simulink model "EMG_DR_E2E_pipeline_simulink"  (R2025a)
settings: Solver=FixedStepAuto  StartTime=0.0  StopTime=inf  FixedStep=0.001  RelTol=1e-3
undefined symbols (not defined in the file or in its folder): magnitude
libraries: slpidlib x4, instrumentseriallib x2, sim3dlib x1, uavsim3dlib x1, deeplib x1
settings Model: Creator=user  LastModifiedBy=82102

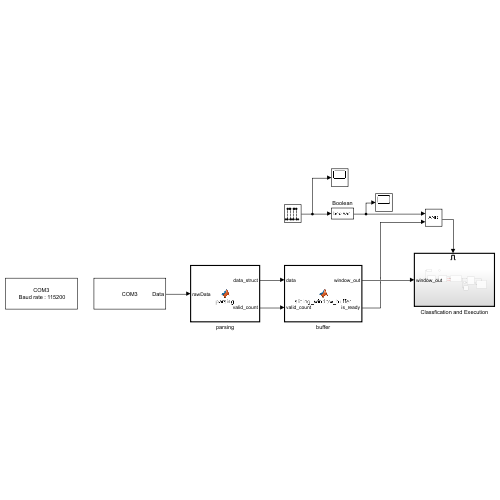
[thumbnail: Simulink's stored preview of the top-level diagram]
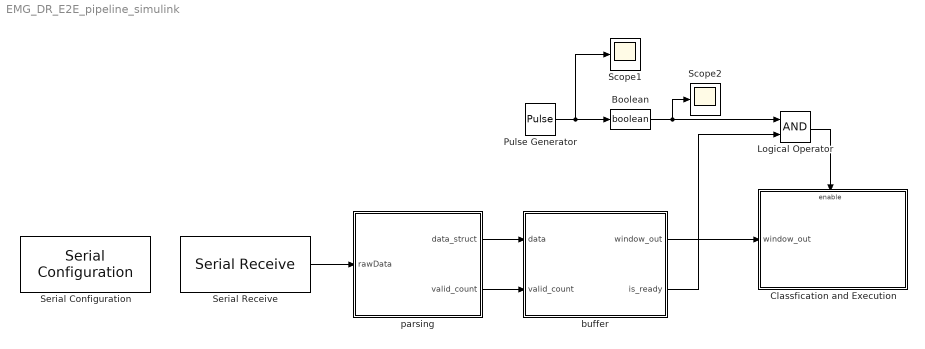
== system EMG_DR_E2E_pipeline_simulink ==
  Boolean : DataTypeConversion  OutDataTypeStr=boolean  SaturateOnIntegerOverflow=off  RndMeth=Floor
  Classfication and Execution : Subsystem  TreatAsAtomicUnit=on
  Logical Operator : Logic  AllPortsSameDT=off  OutDataTypeStr=boolean
  Pulse Generator : DiscretePulseGenerator  Period=100  SampleTime=0.001
  Scope1 : Scope
      settings: ActiveDisplayYMinimum=-1.4E-5  ActiveDisplayYMaximum=1.9E-5
  Scope2 : Scope
      settings: ActiveDisplayYMinimum=-2.3E-6  ActiveDisplayYMaximum=2.1E-6  DataLoggingVariableName=ScopeData2
  Serial Configuration : instrumentseriallib/Serial Configuration  Priority=-200000  PortSel=COM3  Port=COM3  ComPort=COM3  BaudRate=115200  DataBits=8  Parity=none  StopBits=1  ByteOrder=little-endian  FlowControl=none  Timeout=10  SimulateUsing=Interpreted execution  BlockInModel=on  aMode=1
  Serial Receive : instrumentseriallib/Serial Receive  Priority=1  PortSel=COM3  Port=COM3  ComPort=COM3  DataType=uint8  SaveDataType=uint8  ToggleHeader=off  Header=[]  ToggleDataSize=on  DataSize=[1 27]  ToggleTerminator=off  Terminator=<none>  CustomTerminator=[]  InputFormat=Column major  EnableBlockingMode=on  ActionDataUnavailable=Output last received value  ActionWhenDataUnavailable=Output last received value  CustomValue=0  SampleTime=0.001  SimulateUsing=Interpreted execution  BlockInModel=on  aMode=1  LibraryInUse=instrumentlib
  buffer : MATLAB Function  TreatAsAtomicUnit=on
  parsing : MATLAB Function  TreatAsAtomicUnit=on  SystemSampleTime=0.001
  wires:
  Serial Receive/1 -> parsing/1(rawData)
  parsing/1(data_struct) -> buffer/1(data)
  parsing/2(valid_count) -> buffer/2(valid_count)
  Pulse Generator/1 -> Boolean/1, Scope1/1
  Boolean/1 -> Logical Operator/1, Scope2/1
  buffer/1(window_out) -> Classfication and Execution/1(window_out)
  Logical Operator/1 -> Classfication and Execution/Enable
  buffer/2(is_ready) -> Logical Operator/2

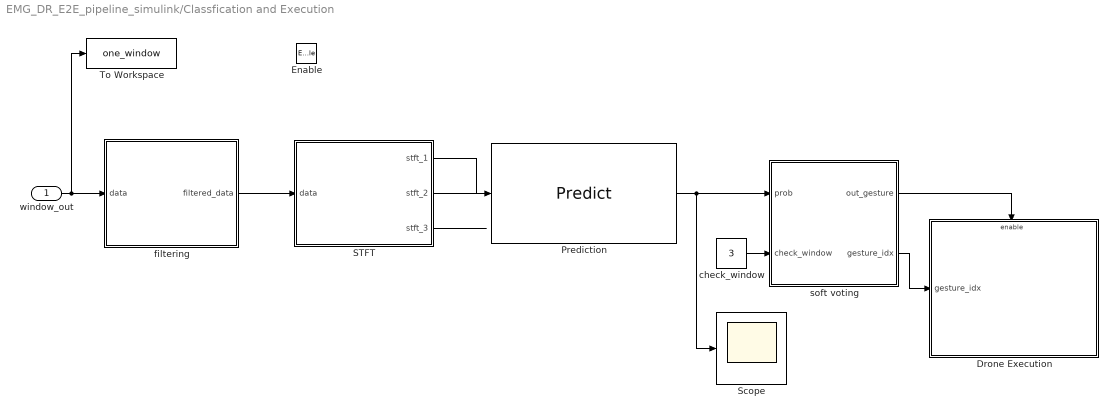
== system EMG_DR_E2E_pipeline_simulink/Classfication and Execution ==
  window_out : Inport
  Enable : EnablePort
  Drone Execution : Subsystem  TreatAsAtomicUnit=on
  Prediction : deeplib/Predict  Network=Network from MAT-file  NetworkFunction=squeezenet  NetworkFilePath=C:\Users\user\Desktop\MATLAB\model\trained_model_3ch_lstm.mat  MiniBatchSize=1  InputDataFormats={'',''}  Predictions=on  Activations={}  ForceInterpretedSim=off  EnableDLNetwork=on  LastKnownNetworkFilePath=''  LastKnownNetworkTimeStamp=''
  STFT : MATLAB Function  TreatAsAtomicUnit=on
  Scope : Scope
      settings: ActiveDisplayYMinimum=-0.125  ActiveDisplayYMaximum=1.125
  To Workspace : ToWorkspace  VariableName=one_window  SampleTime=-1
  check_window : Constant  Value=3
  filtering : MATLAB Function  TreatAsAtomicUnit=on
  soft voting : MATLAB Function  TreatAsAtomicUnit=on
  wires:
  check_window/1 -> soft voting/2(check_window)
  filtering/1(filtered_data) -> STFT/1(data)
  STFT/1(stft_1) -> Prediction/1
  Prediction/1 -> soft voting/1(prob), Scope/1
  window_out/1 -> To Workspace/1, filtering/1(data)
  soft voting/1(out_gesture) -> Drone Execution/Enable
  soft voting/2(gesture_idx) -> Drone Execution/1(gesture_idx)
  STFT/2(stft_2) -> ?
  STFT/3(stft_3) -> ?

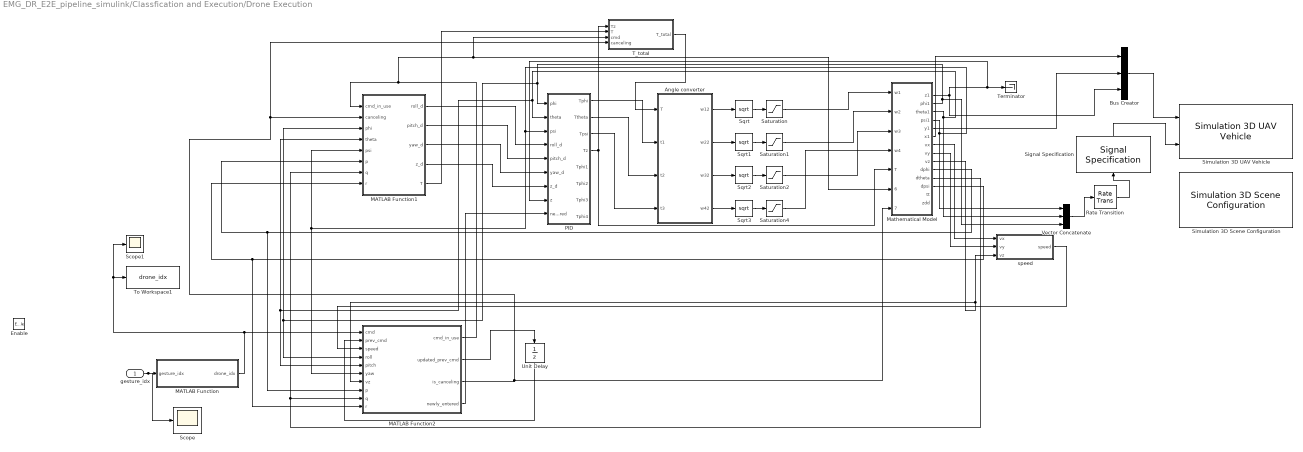
== system EMG_DR_E2E_pipeline_simulink/Classfication and Execution/Drone Execution ==
  gesture_idx : Inport
  Enable : EnablePort
  Angle converter : MATLAB Function  TreatAsAtomicUnit=on
  Bus Creator : BusCreator  Inputs=3
  MATLAB Function : MATLAB Function  TreatAsAtomicUnit=on
  MATLAB Function1 : MATLAB Function  TreatAsAtomicUnit=on
  MATLAB Function2 : MATLAB Function  TreatAsAtomicUnit=on
  Mathematical Model : Subsystem
  PID : Subsystem
  Rate Transition : RateTransition  Deterministic=off  OutPortSampleTime=0.01
  Saturation{,1..2,4} (4 alike) : Saturate  UpperLimit=8000  LowerLimit=0
  Scope : Scope
  Scope1 : Scope
      settings: ActiveDisplayYMinimum=0  ActiveDisplayYMaximum=9
  Signal Specification : SignalSpecification  OutDataTypeStr=double  Dimensions=[1 3]  SampleTime=0.01
  Simulation 3D Scene Configuration : sim3dlib/Simulation 3D Scene Configuration  Priority=0  ProjectFormat=Default Scenes  SceneDesc=US city block  ProjectName=C:\Program Files\MATLAB\R2025a\toolbox\shared\sim3d_projects\automotive_project_windows\UE\WindowsNoEditor\VehicleSimulation.exe  ScenePath=/Game/Maps/USCityBlock  EnableOpenDRIVE=off  vehTagList={'Scene Origin'}  vehTag=Scene Origin  AttachedCameraRelativeTranslation=[0 0 0]  FreeCameraDefaultInitialTranslation=[-6, 0, 2]  AttachedCameraRelativeRotation=[0 0 0]  FreeCameraDefaultInitialRotation=[0, -15, 0]  ViewpointName=Custom  FreeCameraInitialTranslation=[0, 0, 0]  ViewpointTranslation=[0 0 0]  FreeCameraInitialRotation=[0, 0, 0]  ViewpointRotation=[0 0 0]  OpVisEn=off  Ts=0.01  EnableWindow=on  EnableRemoteAccess=off  EnableWeather=off  SunAzimuth=90  SunAltitude=40.0  EnableGeospatialSun=off  Latitude=0  Longitude=0  Date=2023-01-01  Time=10:30:00  GeoTimeZone=-5.0  SunDaylightSaving=off  wind=1  clouds=10  EnableVolumetricClouds=off  CloudCoverage=0  CloudAltitude=6  fog=0  rain=0  RaindropsEffect=off  SnowDensity=0  EnableGeospatial=off  TilesetSource=Earth terrain  UseTrueOrigin=off  OriginHeight=200  OriginLatitude=40.744652  OriginLongitude=-73.988864  MapStyle=Aerial  AdditionalAssetIDs=[]  UseAdvancedSunSky=off  SolarTime=11  TimeZone=-5  Day=21  Month=9  Year=2022  UseDaylightSavingTime=on  DSTStartDay=10  DSTStartMonth=3  DSTEndDay=3  DSTEndMonth=11  DSTSwitchHour=2  sensorTag=MainCamera1  sensorId=1  sensorName=MainCamera1  mountLoc=Origin  offsetFlag=off  tmountOffset=[0, 0, 0]  rmountOffset=[0, 0, 0]  HorizontalResolution=1280  VerticalResolution=720  HorizontalFOV=60  mountPoint=[0 0 0]  mountOrientation=[0 0 0]  aMode=4  ID=1  GeoTrigger=Inactive  ViewNameList={'Custom'}  ViewTranslationList={'[0 0 0]'}  ViewRotationList={'[0 0 0]'}
      settings: LibrarySourceBlock=uavsim3dlib/Simulation 3D Scene Configuration
  Simulation 3D UAV Vehicle : uavsim3dlib/Simulation 3D UAV Vehicle  Priority=-1  Mesh=Quadrotor  MeshPath=/MathWorksUAVContent/UAVs/HexaRotorUAV/HexaRotor.HexaRotor  Color=Red  ActorName=SimulinkVehicle1  UseGlobalFrame=off  InitialTranslation=[0 0 0]  InitialRotation=[0 0 0]  InitialTranslationGlobal=[0 0 0]  InitialGeoOrigin=[0 0 0]  InitialRotationGlobal=[0 0 0]  SampleTime=0.01  ActorType=SimulinkVehicle  ID=1  aMode=4  ActorTag=SimulinkVehicle1
  Sqrt{,1..3} (4 alike) : Sqrt
  T_total : MATLAB Function  TreatAsAtomicUnit=on
  Terminator : Terminator
  To Workspace1 : ToWorkspace  VariableName=drone_idx  SaveFormat=Timeseries  SampleTime=-1
      settings: Save2DSignal=2-D array (concatenate along first dimension)
  Unit Delay : UnitDelay  SampleTime=-1  HasFrameUpgradeWarning=on
  Vector Concatenate : Concatenate  NumInputs=3
  speed : Subsystem
  wires:
  Saturation1/1 -> Mathematical Model/2(w2)
  Angle converter/3(w32) -> Sqrt2/1
  PID/3(Tpsi) -> Angle converter/4(t3)
  Vector Concatenate/1 -> Rate Transition/1
  MATLAB Function1/1(roll_d) -> PID/4(roll_d)
  Bus Creator/1 -> Simulation 3D UAV Vehicle/1
  Mathematical Model/9(vz) -> MATLAB Function2/7(vz), speed/3(vz)
  Mathematical Model/5(y1) -> Bus Creator/2
  MATLAB Function2/1(cmd_in_use) -> MATLAB Function1/1(cmd_in_use), T_total/3(cmd), Mathematical Model/6(cmd_in_use)
  MATLAB Function1/5(T) -> T_total/2(T)
  speed/1(speed) -> MATLAB Function2/3(speed)
  Sqrt2/1 -> Saturation2/1
  Angle converter/2(w22) -> Sqrt1/1
  Saturation/1 -> Mathematical Model/1(w1)
  Mathematical Model/7(vx) -> speed/1(vx)
  PID/2(Ttheta) -> Angle converter/3(t2)
  Saturation4/1 -> Mathematical Model/4(w4)
  MATLAB Function2/3(is_canceling) -> T_total/4(canceling), MATLAB Function1/2(canceling), Mathematical Model/7(is_canceling)
  Saturation2/1 -> Mathematical Model/3(w3)
  MATLAB Function2/2(updated_prev_cmd) -> Unit Delay/1
  Mathematical Model/8(vy) -> speed/2(vy)
  Sqrt/1 -> Saturation/1
  Mathematical Model/6(x1) -> Bus Creator/1
  PID/1(Tphi) -> Angle converter/2(t1)
  MATLAB Function1/3(yaw_d) -> PID/6(yaw_d)
  Angle converter/1(w12) -> Sqrt/1
  Sqrt3/1 -> Saturation4/1
  Signal Specification/1 -> Simulation 3D UAV Vehicle/2
  MATLAB Function2/4(newly_entered) -> PID/9(newly_entered)
  MATLAB Function1/2(pitch_d) -> PID/5(pitch_d)
  Mathematical Model/12(dpsi) -> MATLAB Function1/8(r), MATLAB Function2/10(r)
  Rate Transition/1 -> Signal Specification/1
  Sqrt1/1 -> Saturation1/1
  T_total/1(T_total) -> Angle converter/1(T)
  Angle converter/4(w42) -> Sqrt3/1
  Mathematical Model/1(z1) -> PID/8(z), Terminator/1, Bus Creator/3
  Mathematical Model/3(theta1) -> Vector Concatenate/2, PID/2(theta), MATLAB Function1/4(theta), MATLAB Function2/5(pitch)
  Mathematical Model/4(psi1) -> Vector Concatenate/1, MATLAB Function1/5(psi), MATLAB Function2/6(yaw), PID/3(psi)
  Mathematical Model/10(dphi) -> MATLAB Function1/6(p), MATLAB Function2/8(p)
  Mathematical Model/2(phi1) -> MATLAB Function1/3(phi), MATLAB Function2/4(roll), PID/1(phi), Vector Concatenate/3
  MATLAB Function1/4(z_d) -> PID/7(z_d)
  PID/4(Tz) -> T_total/1(Tz), Mathematical Model/5(T)
  Unit Delay/1 -> MATLAB Function2/2(prev_cmd)
  Mathematical Model/11(dtheta) -> MATLAB Function2/9(q), MATLAB Function1/7(q)
  gesture_idx/1 -> Scope/1, MATLAB Function/1(gesture_idx)
  MATLAB Function/1(drone_idx) -> MATLAB Function2/1(cmd), Scope1/1, To Workspace1/1

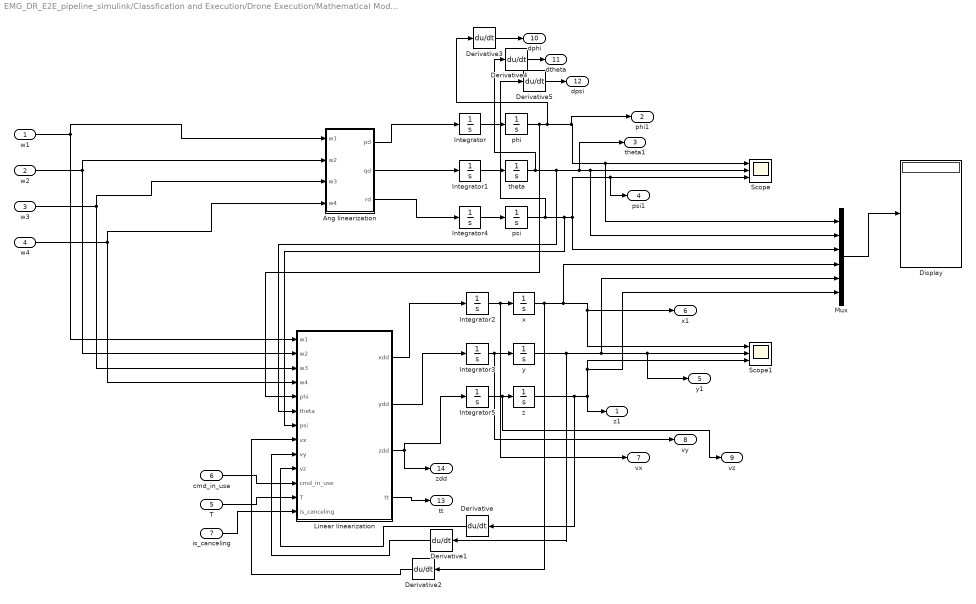
== system EMG_DR_E2E_pipeline_simulink/Classfication and Execution/Drone Execution/Mathematical Model ==
  w1 : Inport
  w2 : Inport  Port=2
  w3 : Inport  Port=3
  w4 : Inport  Port=4
  T : Inport  Port=5
  cmd_in_use : Inport  Port=6
  is_canceling : Inport  Port=7
  Ang linearization : MATLAB Function  TreatAsAtomicUnit=on
  Derivative : Derivative  CoefficientInTFapproximation=0.01
  Derivative1 : Derivative  CoefficientInTFapproximation=0.01
  Derivative2 : Derivative  CoefficientInTFapproximation=0.01
  Derivative3 : Derivative
  Derivative4 : Derivative
  Derivative5 : Derivative
  Display : Display
  Integrator{,1..5} (6 alike) : Integrator
  Linear linearization : MATLAB Function  TreatAsAtomicUnit=on
  Mux : Mux  Inputs=6
  Scope : Scope  NumInputPorts=3
      settings: ActiveDisplayYMinimum=-1  ActiveDisplayYMaximum=1
  Scope1 : Scope  NumInputPorts=3
      settings: ActiveDisplayYMinimum=-3.8299013315849712E+14  ActiveDisplayYMaximum=3.446911198426474E+15
  phi : Integrator
  psi : Integrator
  theta : Integrator
  x : Integrator
  y : Integrator
  z : Integrator
  z1 : Outport
  phi1 : Outport  Port=2
  theta1 : Outport  Port=3
  psi1 : Outport  Port=4
  y1 : Outport  Port=5
  x1 : Outport  Port=6
  vx : Outport  Port=7
  vy : Outport  Port=8
  vz : Outport  Port=9
  dphi : Outport  Port=10
  dtheta : Outport  Port=11
  dpsi : Outport  Port=12
  tt : Outport  Port=13
  zdd : Outport  Port=14
  wires:
  w3/1 -> Ang linearization/3(w3), Linear linearization/3(w3)
  w4/1 -> Ang linearization/4(w4), Linear linearization/4(w4)
  w1/1 -> Ang linearization/1(w1), Linear linearization/1(w1)
  Integrator5/1 -> vz/1, z/1
  Ang linearization/2(qd) -> Integrator1/1
  psi/1 -> Derivative5/1, Linear linearization/7(psi), psi1/1, Scope/3, Mux/3
  Mux/1 -> Display/1
  Integrator4/1 -> psi/1
  w2/1 -> Ang linearization/2(w2), Linear linearization/2(w2)
  Ang linearization/3(rd) -> Integrator4/1
  Linear linearization/2(ydd) -> Integrator3/1
  theta/1 -> Derivative4/1, Linear linearization/6(theta), theta1/1, Mux/2, Scope/2
  Linear linearization/3(zdd) -> Integrator5/1, zdd/1
  phi/1 -> Linear linearization/5(phi), Derivative3/1, phi1/1, Mux/1, Scope/1
  Integrator2/1 -> vx/1, x/1
  Integrator3/1 -> vy/1, y/1
  Linear linearization/1(xdd) -> Integrator2/1
  Integrator1/1 -> theta/1
  x/1 -> Derivative2/1, Mux/4, Scope1/1, x1/1
  z/1 -> Derivative/1, Mux/6, Scope1/3, z1/1
  Ang linearization/1(pd) -> Integrator/1
  Integrator/1 -> phi/1
  y/1 -> Derivative1/1, Mux/5, y1/1, Scope1/2
  Derivative/1 -> Linear linearization/10(vz)
  Derivative1/1 -> Linear linearization/9(vy)
  Derivative2/1 -> Linear linearization/8(vx)
  Linear linearization/4(tt) -> tt/1
  T/1 -> Linear linearization/12(T)
  cmd_in_use/1 -> Linear linearization/11(cmd_in_use)
  is_canceling/1 -> Linear linearization/13(is_canceling)
  Derivative3/1 -> dphi/1
  Derivative4/1 -> dtheta/1
  Derivative5/1 -> dpsi/1

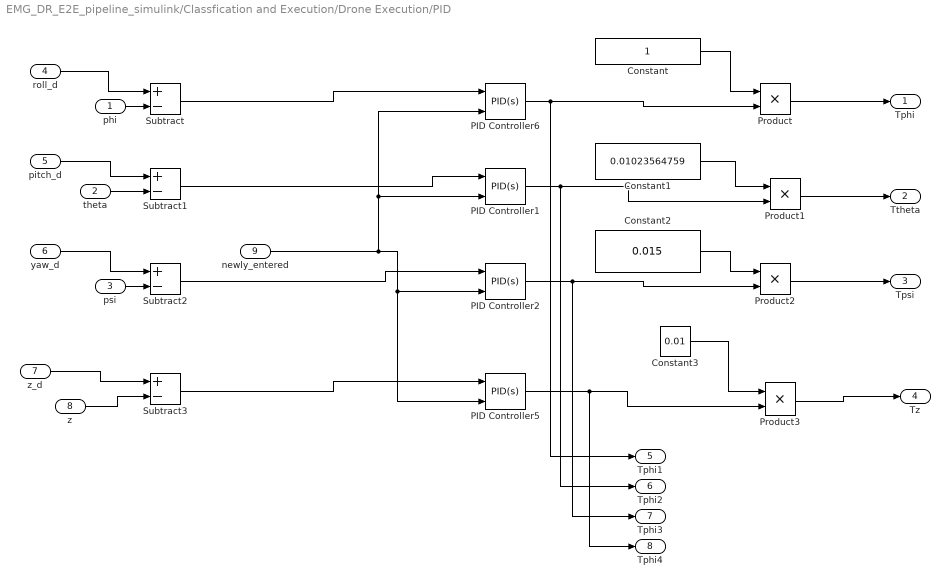
== system EMG_DR_E2E_pipeline_simulink/Classfication and Execution/Drone Execution/PID ==
  phi : Inport
  theta : Inport  Port=2
  psi : Inport  Port=3
  roll_d : Inport  Port=4
  pitch_d : Inport  Port=5
  yaw_d : Inport  Port=6
  z_d : Inport  Port=7
  z : Inport  Port=8
  newly_entered : Inport  Port=9
  Constant : Constant
  Constant1 : Constant  Value=0.01023564759
  Constant2 : Constant  Value=0.015
  Constant3 : Constant  Value=0.01
  PID Controller1 : slpidlib/PID Controller  Controller=PID  Form=Parallel  TimeDomain=Continuous-time  UseExternalTs=off  SampleTime=-1  IntegratorMethod=Forward Euler  FilterMethod=Forward Euler  ControllerParametersSource=internal  P=4.5  I=0.05  UseKiTs=off  D=0.5  UseExternalDerivativeSource=off  N=100  UseFilter=on  TunerSelectOption=Transfer Function Based (PID Tuner App)  InitialConditionSource=internal  InitialConditionForIntegrator=0  InitialConditionForFilter=0  DifferentiatorICPrevScaledInput=0  ExternalReset=rising  TrackingMode=off  Kt=1  LimitOutput=off  SatLimitsSource=internal  UpperSaturationLimit=inf  LowerSaturationLimit=-inf  LinearizeAsGain=on  AntiWindupMode=none  Kb=1  LimitIntegrator=off  UpperIntegratorSaturationLimit=inf  LowerIntegratorSaturationLimit=-inf  POutMin=[]  POutMax=[]  IOutMin=[]  IOutMax=[]  DOutMin=[]  DOutMax=[]  NOutMin=[]  NOutMax=[]  SumOutMin=[]  SumOutMax=[]  SaturationOutMin=[]  SaturationOutMax=[]  PParamMin=[]  PParamMax=[]  IParamMin=[]  IParamMax=[]  DParamMin=[]  DParamMax=[]  NParamMin=[]  NParamMax=[]  KbParamMin=[]  KbParamMax=[]  KtParamMin=[]  KtParamMax=[]  KbOutMin=[]  KbOutMax=[]  KtOutMin=[]  KtOutMax=[]  IntegratorOutMin=[]  IntegratorOutMax=[]  FilterOutMin=[]  FilterOutMax=[]  SumI1OutMin=[]  SumI1OutMax=[]  SumI2OutMin=[]  SumI2OutMax=[]  SumI3OutMin=[]  SumI3OutMax=[]  SumI4OutMin=[]  SumI4OutMax=[]  SumDOutMin=[]  SumDOutMax=[]  DifferentiatorOutMin=[]  DifferentiatorOutMax=[]  FilterDiffOutCoefMin=[]  FilterDiffOutCoefMax=[]  ReciprocalOutMin=[]  ReciprocalOutMax=[]  SumDenOutMin=[]  SumDenOutMax=[]  SumNumOutMin=[]  SumNumOutMax=[]  DivideOutMin=[]  DivideOutMax=[]  UdiffTsProdOutMin=[]  UdiffTsProdOutMax=[]  NTsProdOutMin=[]  NTsProdOutMax=[]  UintegralTsProdOutMin=[]  UintegralTsProdOutMax=[]  UngainTsProdOutMin=[]  UngainTsProdOutMax=[]  ClampingZeroOutDataTypeStr=Inherit: Inherit via back propagation  ClampingZeroOutMin=[]  ClampingZeroOutMax=[]  FilterDenConstantOutDataTypeStr=Inherit: Inherit via back propagation  FilterDenConstantOutMin=[]  FilterDenConstantOutMax=[]  PCopyOutDataTypeStr=Inherit: Inherit via back propagation  PCopyOutMin=[]  PCopyOutMax=[]  NCopyOutDataTypeStr=Inherit: Inherit via back propagation  NCopyOutMin=[]  NCopyOutMax=[]  IntegratorContinuousStateAttributes=''  IntegratorStateMustResolveToSignalObject=off  IntegratorRTWStateStorageClass=Auto  FilterContinuousStateAttributes=''  FilterStateMustResolveToSignalObject=off  FilterRTWStateStorageClass=Auto  ParallelPVariant=InternalParameters  IdealPVariant=Disabled  IVariant=InternalParameters  DVariant=InternalParameters  IntegratorVariant=Continuous  SatVariant=Disabled  AWVariant=Passthrough  PCopyVariant=Disabled  TRVariant=Disabled  FdbkBlocksVariant=Forward  IdealPFdbkVariant=Disabled  SatFdbkVariant=Disabled  DerivativeFilterVariant=ContFilter  NVariant=InternalParameters  NCopyVariant=Disabled  FilterICVariant=InternalICsFilter  IntegratorICVariant=InternalICs  ExternalResetVariant=ExternalReset  TRSumVariant=Passthrough  SumFdbkVariant=Disabled  SumVariant=Sum_PID  TsampFilterVariant=InternalTs  TsampNgainVariant=Passthrough  TsampIntegralVariant=Disabled_SignalSpec  ExternalSaturationOutDataTypeStr=Inherit: Same as second input  DerivativeSourceVariant=ErrorSignal  PreIntVariant=InternalPreInt
  PID Controller2 : slpidlib/PID Controller  Controller=PID  Form=Parallel  TimeDomain=Continuous-time  UseExternalTs=off  SampleTime=-1  IntegratorMethod=Forward Euler  FilterMethod=Forward Euler  ControllerParametersSource=internal  P=2.0  I=0.1  UseKiTs=off  D=0.3  UseExternalDerivativeSource=off  N=100  UseFilter=on  TunerSelectOption=Transfer Function Based (PID Tuner App)  InitialConditionSource=internal  InitialConditionForIntegrator=0  InitialConditionForFilter=0  DifferentiatorICPrevScaledInput=0  ExternalReset=rising  TrackingMode=off  Kt=1  LimitOutput=off  SatLimitsSource=internal  UpperSaturationLimit=inf  LowerSaturationLimit=-inf  LinearizeAsGain=on  AntiWindupMode=none  Kb=1  LimitIntegrator=off  UpperIntegratorSaturationLimit=inf  LowerIntegratorSaturationLimit=-inf  POutMin=[]  POutMax=[]  IOutMin=[]  IOutMax=[]  DOutMin=[]  DOutMax=[]  NOutMin=[]  NOutMax=[]  SumOutMin=[]  SumOutMax=[]  SaturationOutMin=[]  SaturationOutMax=[]  PParamMin=[]  PParamMax=[]  IParamMin=[]  IParamMax=[]  DParamMin=[]  DParamMax=[]  NParamMin=[]  NParamMax=[]  KbParamMin=[]  KbParamMax=[]  KtParamMin=[]  KtParamMax=[]  KbOutMin=[]  KbOutMax=[]  KtOutMin=[]  KtOutMax=[]  IntegratorOutMin=[]  IntegratorOutMax=[]  FilterOutMin=[]  FilterOutMax=[]  SumI1OutMin=[]  SumI1OutMax=[]  SumI2OutMin=[]  SumI2OutMax=[]  SumI3OutMin=[]  SumI3OutMax=[]  SumI4OutMin=[]  SumI4OutMax=[]  SumDOutMin=[]  SumDOutMax=[]  DifferentiatorOutMin=[]  DifferentiatorOutMax=[]  FilterDiffOutCoefMin=[]  FilterDiffOutCoefMax=[]  ReciprocalOutMin=[]  ReciprocalOutMax=[]  SumDenOutMin=[]  SumDenOutMax=[]  SumNumOutMin=[]  SumNumOutMax=[]  DivideOutMin=[]  DivideOutMax=[]  UdiffTsProdOutMin=[]  UdiffTsProdOutMax=[]  NTsProdOutMin=[]  NTsProdOutMax=[]  UintegralTsProdOutMin=[]  UintegralTsProdOutMax=[]  UngainTsProdOutMin=[]  UngainTsProdOutMax=[]  ClampingZeroOutDataTypeStr=Inherit: Inherit via back propagation  ClampingZeroOutMin=[]  ClampingZeroOutMax=[]  FilterDenConstantOutDataTypeStr=Inherit: Inherit via back propagation  FilterDenConstantOutMin=[]  FilterDenConstantOutMax=[]  PCopyOutDataTypeStr=Inherit: Inherit via back propagation  PCopyOutMin=[]  PCopyOutMax=[]  NCopyOutDataTypeStr=Inherit: Inherit via back propagation  NCopyOutMin=[]  NCopyOutMax=[]  IntegratorContinuousStateAttributes=''  IntegratorStateMustResolveToSignalObject=off  IntegratorRTWStateStorageClass=Auto  FilterContinuousStateAttributes=''  FilterStateMustResolveToSignalObject=off  FilterRTWStateStorageClass=Auto  ParallelPVariant=InternalParameters  IdealPVariant=Disabled  IVariant=InternalParameters  DVariant=InternalParameters  IntegratorVariant=Continuous  SatVariant=Disabled  AWVariant=Passthrough  PCopyVariant=Disabled  TRVariant=Disabled  FdbkBlocksVariant=Forward  IdealPFdbkVariant=Disabled  SatFdbkVariant=Disabled  DerivativeFilterVariant=ContFilter  NVariant=InternalParameters  NCopyVariant=Disabled  FilterICVariant=InternalICsFilter  IntegratorICVariant=InternalICs  ExternalResetVariant=ExternalReset  TRSumVariant=Passthrough  SumFdbkVariant=Disabled  SumVariant=Sum_PID  TsampFilterVariant=InternalTs  TsampNgainVariant=Passthrough  TsampIntegralVariant=Disabled_SignalSpec  ExternalSaturationOutDataTypeStr=Inherit: Same as second input  DerivativeSourceVariant=ErrorSignal  PreIntVariant=InternalPreInt
  PID Controller5 : slpidlib/PID Controller  Controller=PID  Form=Parallel  TimeDomain=Continuous-time  UseExternalTs=off  SampleTime=-1  IntegratorMethod=Forward Euler  FilterMethod=Forward Euler  ControllerParametersSource=internal  P=5  I=3  UseKiTs=off  D=0  UseExternalDerivativeSource=off  N=100  UseFilter=on  TunerSelectOption=Transfer Function Based (PID Tuner App)  InitialConditionSource=internal  InitialConditionForIntegrator=0  InitialConditionForFilter=0  DifferentiatorICPrevScaledInput=0  ExternalReset=rising  TrackingMode=off  Kt=1  LimitOutput=off  SatLimitsSource=internal  UpperSaturationLimit=inf  LowerSaturationLimit=-inf  LinearizeAsGain=on  AntiWindupMode=none  Kb=1  LimitIntegrator=off  UpperIntegratorSaturationLimit=inf  LowerIntegratorSaturationLimit=-inf  POutMin=[]  POutMax=[]  IOutMin=[]  IOutMax=[]  DOutMin=[]  DOutMax=[]  NOutMin=[]  NOutMax=[]  SumOutMin=[]  SumOutMax=[]  SaturationOutMin=[]  SaturationOutMax=[]  PParamMin=[]  PParamMax=[]  IParamMin=[]  IParamMax=[]  DParamMin=[]  DParamMax=[]  NParamMin=[]  NParamMax=[]  KbParamMin=[]  KbParamMax=[]  KtParamMin=[]  KtParamMax=[]  KbOutMin=[]  KbOutMax=[]  KtOutMin=[]  KtOutMax=[]  IntegratorOutMin=[]  IntegratorOutMax=[]  FilterOutMin=[]  FilterOutMax=[]  SumI1OutMin=[]  SumI1OutMax=[]  SumI2OutMin=[]  SumI2OutMax=[]  SumI3OutMin=[]  SumI3OutMax=[]  SumI4OutMin=[]  SumI4OutMax=[]  SumDOutMin=[]  SumDOutMax=[]  DifferentiatorOutMin=[]  DifferentiatorOutMax=[]  FilterDiffOutCoefMin=[]  FilterDiffOutCoefMax=[]  ReciprocalOutMin=[]  ReciprocalOutMax=[]  SumDenOutMin=[]  SumDenOutMax=[]  SumNumOutMin=[]  SumNumOutMax=[]  DivideOutMin=[]  DivideOutMax=[]  UdiffTsProdOutMin=[]  UdiffTsProdOutMax=[]  NTsProdOutMin=[]  NTsProdOutMax=[]  UintegralTsProdOutMin=[]  UintegralTsProdOutMax=[]  UngainTsProdOutMin=[]  UngainTsProdOutMax=[]  ClampingZeroOutDataTypeStr=Inherit: Inherit via back propagation  ClampingZeroOutMin=[]  ClampingZeroOutMax=[]  FilterDenConstantOutDataTypeStr=Inherit: Inherit via back propagation  FilterDenConstantOutMin=[]  FilterDenConstantOutMax=[]  PCopyOutDataTypeStr=Inherit: Inherit via back propagation  PCopyOutMin=[]  PCopyOutMax=[]  NCopyOutDataTypeStr=Inherit: Inherit via back propagation  NCopyOutMin=[]  NCopyOutMax=[]  IntegratorContinuousStateAttributes=''  IntegratorStateMustResolveToSignalObject=off  IntegratorRTWStateStorageClass=Auto  FilterContinuousStateAttributes=''  FilterStateMustResolveToSignalObject=off  FilterRTWStateStorageClass=Auto  ParallelPVariant=InternalParameters  IdealPVariant=Disabled  IVariant=InternalParameters  DVariant=InternalParameters  IntegratorVariant=Continuous  SatVariant=Disabled  AWVariant=Passthrough  PCopyVariant=Disabled  TRVariant=Disabled  FdbkBlocksVariant=Forward  IdealPFdbkVariant=Disabled  SatFdbkVariant=Disabled  DerivativeFilterVariant=ContFilter  NVariant=InternalParameters  NCopyVariant=Disabled  FilterICVariant=InternalICsFilter  IntegratorICVariant=InternalICs  ExternalResetVariant=ExternalReset  TRSumVariant=Passthrough  SumFdbkVariant=Disabled  SumVariant=Sum_PID  TsampFilterVariant=InternalTs  TsampNgainVariant=Passthrough  TsampIntegralVariant=Disabled_SignalSpec  ExternalSaturationOutDataTypeStr=Inherit: Same as second input  DerivativeSourceVariant=ErrorSignal  PreIntVariant=InternalPreInt
  PID Controller6 : slpidlib/PID Controller  Controller=PID  Form=Parallel  TimeDomain=Continuous-time  UseExternalTs=off  SampleTime=-1  IntegratorMethod=Forward Euler  FilterMethod=Forward Euler  ControllerParametersSource=internal  P=4.5  I=0.05  UseKiTs=off  D=0.5  UseExternalDerivativeSource=off  N=100  UseFilter=on  TunerSelectOption=Transfer Function Based (PID Tuner App)  InitialConditionSource=internal  InitialConditionForIntegrator=0  InitialConditionForFilter=0  DifferentiatorICPrevScaledInput=0  ExternalReset=rising  TrackingMode=off  Kt=1  LimitOutput=off  SatLimitsSource=internal  UpperSaturationLimit=inf  LowerSaturationLimit=-inf  LinearizeAsGain=on  AntiWindupMode=none  Kb=1  LimitIntegrator=off  UpperIntegratorSaturationLimit=inf  LowerIntegratorSaturationLimit=-inf  POutMin=[]  POutMax=[]  IOutMin=[]  IOutMax=[]  DOutMin=[]  DOutMax=[]  NOutMin=[]  NOutMax=[]  SumOutMin=[]  SumOutMax=[]  SaturationOutMin=[]  SaturationOutMax=[]  PParamMin=[]  PParamMax=[]  IParamMin=[]  IParamMax=[]  DParamMin=[]  DParamMax=[]  NParamMin=[]  NParamMax=[]  KbParamMin=[]  KbParamMax=[]  KtParamMin=[]  KtParamMax=[]  KbOutMin=[]  KbOutMax=[]  KtOutMin=[]  KtOutMax=[]  IntegratorOutMin=[]  IntegratorOutMax=[]  FilterOutMin=[]  FilterOutMax=[]  SumI1OutMin=[]  SumI1OutMax=[]  SumI2OutMin=[]  SumI2OutMax=[]  SumI3OutMin=[]  SumI3OutMax=[]  SumI4OutMin=[]  SumI4OutMax=[]  SumDOutMin=[]  SumDOutMax=[]  DifferentiatorOutMin=[]  DifferentiatorOutMax=[]  FilterDiffOutCoefMin=[]  FilterDiffOutCoefMax=[]  ReciprocalOutMin=[]  ReciprocalOutMax=[]  SumDenOutMin=[]  SumDenOutMax=[]  SumNumOutMin=[]  SumNumOutMax=[]  DivideOutMin=[]  DivideOutMax=[]  UdiffTsProdOutMin=[]  UdiffTsProdOutMax=[]  NTsProdOutMin=[]  NTsProdOutMax=[]  UintegralTsProdOutMin=[]  UintegralTsProdOutMax=[]  UngainTsProdOutMin=[]  UngainTsProdOutMax=[]  ClampingZeroOutDataTypeStr=Inherit: Inherit via back propagation  ClampingZeroOutMin=[]  ClampingZeroOutMax=[]  FilterDenConstantOutDataTypeStr=Inherit: Inherit via back propagation  FilterDenConstantOutMin=[]  FilterDenConstantOutMax=[]  PCopyOutDataTypeStr=Inherit: Inherit via back propagation  PCopyOutMin=[]  PCopyOutMax=[]  NCopyOutDataTypeStr=Inherit: Inherit via back propagation  NCopyOutMin=[]  NCopyOutMax=[]  IntegratorContinuousStateAttributes=''  IntegratorStateMustResolveToSignalObject=off  IntegratorRTWStateStorageClass=Auto  FilterContinuousStateAttributes=''  FilterStateMustResolveToSignalObject=off  FilterRTWStateStorageClass=Auto  ParallelPVariant=InternalParameters  IdealPVariant=Disabled  IVariant=InternalParameters  DVariant=InternalParameters  IntegratorVariant=Continuous  SatVariant=Disabled  AWVariant=Passthrough  PCopyVariant=Disabled  TRVariant=Disabled  FdbkBlocksVariant=Forward  IdealPFdbkVariant=Disabled  SatFdbkVariant=Disabled  DerivativeFilterVariant=ContFilter  NVariant=InternalParameters  NCopyVariant=Disabled  FilterICVariant=InternalICsFilter  IntegratorICVariant=InternalICs  ExternalResetVariant=ExternalReset  TRSumVariant=Passthrough  SumFdbkVariant=Disabled  SumVariant=Sum_PID  TsampFilterVariant=InternalTs  TsampNgainVariant=Passthrough  TsampIntegralVariant=Disabled_SignalSpec  ExternalSaturationOutDataTypeStr=Inherit: Same as second input  DerivativeSourceVariant=ErrorSignal  PreIntVariant=InternalPreInt
  Product{,1..3} (4 alike) : Product
  Subtract{,1..3} (4 alike) : Sum  Inputs=+-
  Tphi : Outport
  Ttheta : Outport  Port=2
  Tpsi : Outport  Port=3
  Tz : Outport  Port=4
  Tphi1 : Outport  Port=5
  Tphi2 : Outport  Port=6
  Tphi3 : Outport  Port=7
  Tphi4 : Outport  Port=8
  wires:
  phi/1 -> Subtract/2
  Subtract/1 -> PID Controller6/1
  Subtract1/1 -> PID Controller1/1
  Subtract2/1 -> PID Controller2/1
  theta/1 -> Subtract1/2
  psi/1 -> Subtract2/2
  roll_d/1 -> Subtract/1
  pitch_d/1 -> Subtract1/1
  yaw_d/1 -> Subtract2/1
  Product2/1 -> Tpsi/1
  Product1/1 -> Ttheta/1
  Product/1 -> Tphi/1
  Constant/1 -> Product/1
  Constant2/1 -> Product2/1
  Constant1/1 -> Product1/1
  PID Controller6/1 -> Tphi1/1, Product/2
  PID Controller1/1 -> Tphi2/1, Product1/2
  PID Controller2/1 -> Tphi3/1, Product2/2
  Constant3/1 -> Product3/1
  Product3/1 -> Tz/1
  PID Controller5/1 -> Tphi4/1, Product3/2
  Subtract3/1 -> PID Controller5/1
  z_d/1 -> Subtract3/1
  z/1 -> Subtract3/2
  newly_entered/1 -> PID Controller5/2, PID Controller2/2, PID Controller1/2, PID Controller6/2

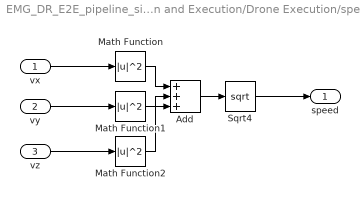
== system EMG_DR_E2E_pipeline_simulink/Classfication and Execution/Drone Execution/speed ==
  vx : Inport
  vy : Inport  Port=2
  vz : Inport  Port=3
  Add : Sum  Inputs=+++
  Math Function : Math  Operator=magnitude^2
  Math Function1 : Math  Operator=magnitude^2
  Math Function2 : Math  Operator=magnitude^2
  Sqrt4 : Sqrt
  speed : Outport
  wires:
  Math Function2/1 -> Add/3
  Math Function/1 -> Add/1
  Math Function1/1 -> Add/2
  Add/1 -> Sqrt4/1
  Sqrt4/1 -> speed/1
  vy/1 -> Math Function1/1
  vz/1 -> Math Function2/1
  vx/1 -> Math Function/1

== matlab function EMG_DR_E2E_pipeline_simulink/Classfication and Execution/Drone Execution/MATLAB Function1 ==
  settings: updateMethod=DISCRETE  sampleTime=0.01
  data: cmd_in_use input; roll_d output; pitch_d output; yaw_d output; z_d output; canceling input; T output; phi input; theta input; psi input; p input; q input; r input
function [roll_d, pitch_d, yaw_d, z_d, T] = ...
    cmdDispatcher(cmd_in_use, canceling, phi, theta, psi, p, q, r)

roll_d = 0;
pitch_d = 0;
yaw_d = 0;
z_d = 0;
T = 0;

% 시작 명령 처리
if cmd_in_use == 0
    return;
end

hover_z = 0;
hover_T = 0.6;
move_T = 13;
ascend_T = 15;
descend_T = 11.0;


% 보정 상태 처리
if canceling == 1
    z_d     = hover_z;

    % === 흔들림 피드백 보정 추가 ===
    Kp_phi2 = 7.0;   % 기울기 비례 이득 (롤)
    Kp_theta2 = 7.0; % 기울기 비례 이득 (피치)
    Kp_yaw2 = 7.0;

    % 새로 추가: 관성 감쇠용 D항
    Kd_phi2 = 0.05;
    Kd_theta2 = 0.05;
    Kd_yaw2 = 0.05;

    roll_d  = -(Kp_phi2 * phi + Kd_phi2 * p);
    pitch_d = -(Kp_theta2 * theta + Kd_theta2 * q);
    yaw_d   = -(Kp_yaw2 * psi + Kd_yaw2 * r);


    % z축 성분 기반 추력 보강
    % canceling == 1인 경우
    z_axis_projection = max(cos(phi)*cos(theta), 0.4);
    T = hover_T / z_axis_projection;
    
    % 추가로 안정적 범위 안에 고정
    T = min(max(T, hover_T), move_T);  % T ∈ [hover_T, move_T]
    return;
end

% === 흔들림 피드백 보정 추가 ===
Kp_phi = 1.5;   % 기울기 비례 이득 (롤)
Kp_theta = 1.5; % 기울기 비례 이득 (피치)
Kp_yaw = 1.5;

% 동작 처리
switch cmd_in_use
    
        case 1  % 전진
        pitch_d = 0.5 - Kp_theta * theta;
        roll_d  = -Kp_phi * phi;
        yaw_d   = -Kp_yaw * psi;
        z_d = hover_z;
        T = move_T;
    
    case 2  % 후진
        pitch_d = -0.5 - Kp_theta * theta;
        roll_d  = -Kp_phi * phi;
        yaw_d   = -Kp_yaw * psi;
        z_d = hover_z;
        T = move_T;
    
    case 3  % 상승
        pitch_d = -Kp_theta * theta;
        roll_d  = -Kp_phi * phi;
        yaw_d   = -Kp_yaw * psi;
        z_d = hover_z + 0.5;
        T = ascend_T;
    
    case 4  % 하강
        pitch_d = -Kp_theta * theta;
        roll_d  = -Kp_phi * phi;
        yaw_d   = -Kp_yaw * psi;
        z_d = hover_z - 0.5;
        T = descend_T;
    
    case 5  % 좌
        roll_d = -0.6 - Kp_phi * phi;
        pitch_d = -Kp_theta * theta;
        yaw_d   = -Kp_yaw * psi;
        z_d = hover_z;
        T = move_T;
    
    case 6  % 우
        roll_d = 0.6 - Kp_phi * phi;
        pitch_d = -Kp_theta * theta;
        yaw_d   = -Kp_yaw * psi;
        z_d = hover_z;
        T = move_T;
    
    case 7  % 정지
        pitch_d = -Kp_theta * theta;
        roll_d  = -Kp_phi * phi;
        yaw_d   = -Kp_yaw * psi;
        z_d = hover_z;
        T = hover_T;
    otherwise
        roll_d = 0;
        pitch_d = 0;
        yaw_d = 0;
        z_d = hover_z;
        T = hover_T;
end

end

== matlab function EMG_DR_E2E_pipeline_simulink/Classfication and Execution/Drone Execution/MATLAB Function2 ==
  settings: updateMethod=DISCRETE
  data: cmd input; cmd_in_use output; prev_cmd input; speed input; updated_prev_cmd output; is_canceling output; roll input; pitch input; yaw input; vz input; newly_entered output; p input; q input; r input
function [cmd_in_use, updated_prev_cmd, is_canceling, newly_entered] = CmdFSMManager(cmd, prev_cmd, speed, roll, pitch, yaw, vz,  p, q, r)


eps_speed = 0.01;                 % 속도 허용값 (m/s)
eps_phi_abs = deg2rad(2);         % roll 허용 오차 (±2도)
eps_theta_abs = deg2rad(2);       % pitch 허용 오차 (±2도)
eps_yaw_abs = deg2rad(2);  
vz_threshold = 0.2;  % 상승/하강 판단용 속도 기준

cmd_in_use = 0.0;
updated_prev_cmd = 0.0;
is_canceling = 0.0;


persistent is_canceling_internal cmd_hold prev_speed
% is_canceling_internal: 현재 보정 중 상태인지 여부를 저장
% cmd_hold: 보정 중일 때 실행을 유지해야 할 명령 (이전 명령)
% prev_speed: 이전 시점의 속도 저장

if isempty(is_canceling_internal); is_canceling_internal = 0.0; end
if isempty(cmd_hold);              cmd_hold = prev_cmd;          end
if isempty(prev_speed);            prev_speed = 0;               end

persistent stable_cnt
if isempty(stable_cnt)
    stable_cnt = 0;
end


% 상태 전환 조건
cmd_changed = (cmd ~= prev_cmd);


% === 보정 종료 조건 계산 ===
% 1) 작은 속도, 2) 작은 각도, 3) 각도의 변화량도 충분히 작을 때

if is_canceling_internal
    if abs(speed) < eps_speed && abs(vz) < abs(vz_threshold) && ...
       abs(roll) < eps_phi_abs && abs(pitch) < eps_theta_abs && abs(yaw) < eps_yaw_abs && ...
       abs(p) < 0.02 && abs(q) < 0.02 && abs(r) < 0.02
        stable_cnt = stable_cnt + 1;
    else
        stable_cnt = 0;
    end

    if stable_cnt >= 100  % 100번 연속 만족해야 종료
        is_canceling_internal = 0.0;
        stable_cnt = 0;
    end
end


persistent was_canceling
newly_entered = (is_canceling == 1.0 && was_canceling == 0.0);
newly_entered = logical(newly_entered);
was_canceling = is_canceling;


if cmd_changed && (abs(speed) > eps_speed || abs(vz) > vz_threshold)
% 다음 조건 2개가 함께 만족하면 보정 상태 진입
    % 조건 1) 명령이 변경됨 (cmd ≠ prev_cmd) 
    % 조건 2) 현재 속도가 커야 함 → 즉, 빠르게 움직이는 중일 때만 보정
    is_canceling_internal = 1.0;
    cmd_hold = prev_cmd;  % 이전 명령 기억
    stable_cnt = 0;       % 카운터 초기화
end

% 0번 명령이면 무조건 초기화 모드
if cmd == 0
    is_canceling = 0.0;
    cmd_in_use = 0;
    updated_prev_cmd = 0;
    is_canceling_internal = 0.0;
    cmd_hold = 0;
    prev_speed = 0;
    stable_cnt = 0;
    was_canceling = 0;
    newly_entered = false;
    return;
end




% 출력 명령 결정
% 보정 중이면: cmd_in_use: cmd_hold (이전 명령 유지) / updated_prev_cmd: 그대로 유지
% 보정 중이 아니면: cmd_in_use: 새로운 명령 사용 / updated_prev_cmd: 새로운 명령으로 갱신

if is_canceling_internal == 1.0 
    cmd_in_use = cmd_hold;        % 이전 명령 계속 사용
    updated_prev_cmd = prev_cmd; 
else
    cmd_in_use = cmd;            % 새로운 명령 사용
    updated_prev_cmd = cmd; 
end

is_canceling = is_canceling_internal;


% 상태 저장
prev_speed = speed;

== matlab function EMG_DR_E2E_pipeline_simulink/Classfication and Execution/Drone Execution/T_total ==
  data: Tz input; T_total output; T input; cmd input; canceling input
function T_total  = fcn(Tz, T, cmd, canceling)

if (cmd == 7 || canceling == 1.0)
    % 정지 명령 또는 보정 중에는 PID 제어만 사용
    T_total = Tz;
elseif (cmd == 3 || cmd == 4)
    % 상승/하강 시엔 PID 기반 + 명령 기반 추력을 적당히 섞기
    T_total = 0.6 * T + 0.4 * Tz;
else
    % 나머지는 명령 기반 추력만 사용
    T_total = T;
end

% === 출력 제한 (물리적으로 적절한 범위로 클리핑) ===
T_total = min(max(T_total, 0), 20);  % 필요 시 상한/하한 조절

== matlab function EMG_DR_E2E_pipeline_simulink/Classfication and Execution/Drone Execution/Mathematical Model/Ang linearization ==
  data: w1 input; pd output; w2 input; w3 input; w4 input; qd output; rd output
function [pd,qd,rd] = fcn(w1,w2,w3,w4)

d=0.176777;
ct=8.586e-08;
cq=4.81e-09;
Jxx=0.01023564759;
Jyy=0.01023564759;
Jzz=0.02047129518;

pd=(d*ct*(-w1^2 + w2^2 + w3^2 - w4^2)/(Jxx*1.414));
qd=(d*ct*(-w1^2 - w2^2 + w3^2 + w4^2)/(Jyy*1.414));
rd=(cq*(-w1^2 + w2^2 - w3^2 + w4^2)/Jzz);

== matlab function EMG_DR_E2E_pipeline_simulink/Classfication and Execution/Drone Execution/Mathematical Model/Linear linearization ==
  settings: updateMethod=DISCRETE
  data: w1 input; xdd output; w2 input; w3 input; w4 input; phi input; theta input; psi input; ydd output; zdd output; vx input; vy input; vz input; tt output; cmd_in_use input; T input; is_canceling input
function [xdd, ydd, zdd, tt] = fcn(w1, w2, w3, w4, phi, theta, psi, vx, vy, vz, cmd_in_use, T, is_canceling)

g = 9.81;               % 중력
m = 1.5;                % 드론 질량
ct = 8.586e-08;         % 양력 계수
k_drag = 1.2;           % 공기 저항 계수
v_thresh = 0.001;        % 공기저항 종료 속도 임계값

% 총 추력 계산
tt = ct * (w1^2 + w2^2 + w3^2 + w4^2);
if tt < 1e-6
    tt = 1e-6; 
end

% 본래 기울기 기반 thrust 가속도 계산
xdd_thrust = (phi * sin(psi) + theta * cos(psi)) * tt / m;
ydd_thrust = (theta * sin(phi) - phi * cos(psi)) * tt / m;

persistent last_Tz_override

if isempty(last_Tz_override)
    last_Tz_override = 0;
end

% z축 thrust 가속도 계산
if ~is_canceling && cmd_in_use == 4
    % 하강
    target_zdd = -0.3;
    T_target = m * (g + target_zdd);
    last_Tz_override = T_target - T;
    zdd_thrust = target_zdd;

elseif ~is_canceling && cmd_in_use == 3
    % 상승
    target_zdd = 0.3;
    T_target = m * (g + target_zdd);
    last_Tz_override = T_target - T;
    zdd_thrust = target_zdd;

else
    if tt <= m * g
        zdd_thrust = 0;
    else
        zdd_thrust = (-m * g + tt) / m;
    end
end

% 속도 크기 계산
v_mag = sqrt(vx^2 + vy^2 + vz^2);

K_dvz = 1.5;

%공기 저항력 계산
if v_mag > v_thresh
    drag_x = -k_drag * vx;
    drag_y = -k_drag * vy;
    drag_z = -k_drag * vz;
else
    drag_x = 0;
    drag_y = 0;
    drag_z = 0;
end

% canceling일 때, z축 damping 추가 보강
if is_canceling
    drag_z = drag_z - K_dvz * vz;
end

% 최종 가속도 (Thrust + Drag)
xdd = xdd_thrust + drag_x;
ydd = ydd_thrust + drag_y;
zdd = zdd_thrust + drag_z;

if isnan(tt) || isnan(xdd) || isnan(ydd) || isnan(zdd)
    error("NaN detected in thrust or acceleration calculation.");
end


end

== matlab function EMG_DR_E2E_pipeline_simulink/Classfication and Execution/filtering ==
  data: data input; filtered_data output
function filtered_data = filtering(data)
    persistent zi1 zi2
    persistent b60 a60 b a
    fs = 1000;
    
    if isempty(b60)
        [b60, a60] = butter(2, [55 65] / (fs / 2), 'stop'); 
        [b, a]     = butter(2, [20 450] / (fs / 2), 'bandpass');
    end
    
    if isempty(zi1)
        zi1 = zeros(max(length(a60), length(b60)) - 1, 3);
        zi2 = zeros(max(length(a), length(b)) - 1, 3);
    end
    
    [filtered_data, zi1] = filter(b60, a60, data, zi1);
    [filtered_data, zi2] = filter(b, a, filtered_data, zi2);

== matlab function EMG_DR_E2E_pipeline_simulink/parsing ==
  data: data_struct output double size=[200 3]; rawData input uint8; valid_count output
function [data_struct, valid_count] = parsing(rawData)

    channels = 3;
    Byte = 9;
    HEADER = [170 119 170];
    MAX_LEFT = 1024;
    MAX_PARSED = 200;

    data_struct = zeros(MAX_PARSED, channels);
    valid_count = 0;

    persistent left_data left_length
    if isempty(left_data)
        left_data = zeros(1, MAX_LEFT, 'uint8');
        left_length = 0;
    end

    rawData = [left_data(1:left_length), rawData];
    N = length(rawData);
    i = 1;

    while i <= N - Byte
        if all(rawData(i:i+2) == HEADER)
            if valid_count < MAX_PARSED
                Data = zeros(1, channels);
                for ch = 1:channels
                    idx = i + 2 + 2*(ch - 1) + 1;
                    if idx + 1 <= N
                        val = double(rawData(idx)) * 256 + double(rawData(idx+1));
                        mv = ((val / 4095) * 10.0 - 5.0) * 1000.0;
                        Data(ch) = mv;
                    end
                end
                valid_count = valid_count + 1;
                data_struct(valid_count, :) = Data;
            end
            i = i + Byte;
        else
            i = i + 1;
        end
    end

    leftover = rawData(i:end);
    left_length = length(leftover);
    left_data = zeros(1, MAX_LEFT, 'uint8');
    left_data(1:min(left_length, MAX_LEFT)) = leftover;
end

== matlab function EMG_DR_E2E_pipeline_simulink/Classfication and Execution/STFT ==
  data: data input; stft_1 output; stft_2 output; stft_3 output
function [stft_1, stft_2, stft_3]= feature_extraction(data)

    fs = 1000;
    winLen = round(0.2 * fs);
    overlap = round(0.18 * fs);
    fftLen = 256;
    epsilon = 1e-6;
    fmin = 20;
    fmax = 450;
    channels = 3;
    [~, f, t_, ps] = spectrogram(zeros(fs,1), winLen, overlap, fftLen, fs);
    idx_range = (f>fmin) & (f < fmax);
    freq_bins = 110;
    time_frames = numel(t_);

    stft_tensor = zeros(freq_bins, time_frames, channels);

    for ch = 1:channels
        sig = data(:, ch);
        [~, ~, ~, ps] = spectrogram(sig, winLen, overlap, fftLen, fs);
        ps_db = 10 * log10(abs(ps));
        stft_tensor(:,:,ch) = ps_db(idx_range, :);
    end

    mu = mean(stft_tensor, [1 2]);
    sigma = std(stft_tensor, 0, [1 2]);
    sigma(sigma < epsilon) = 1;

    stft_tensor = (stft_tensor - mu) ./ sigma;
    stft_tensor = reshape(stft_tensor, freq_bins, time_frames, channels, 1);
    stft_1 = stft_tensor(:, :, 1, :);
    stft_2 = stft_tensor(:, :, 2, :);
    stft_3 = stft_tensor(:, :, 3, :);
end

== matlab function EMG_DR_E2E_pipeline_simulink/Classfication and Execution/soft voting ==
  data: out_gesture output; prob input; gesture_idx output; check_window input
function [out_gesture, gesture_idx] = smoothedVoting(prob, check_window)
    
    persistent probs count 
    if isempty(probs)
        probs = zeros(3, 8); % 3개의 예측 결과 저장
        count = 1;
    end

    gesture_idx = 0;      % <-- 초기화
    out_gesture = false; 
    
    count = count + 1;
    probs(mod(count-1,3)+1, :) = prob;
    
    if count > check_window
        sum_prob = sum(probs, 1);              
        norm_prob = sum_prob / norm(sum_prob);
        [~, gesture_idx] = max(norm_prob);
        out_gesture = true; 
        count = 1;
    end
end

== matlab function EMG_DR_E2E_pipeline_simulink/buffer ==
  data: data input; window_out output; valid_count input; is_ready output
function [window_out, is_ready] = sliding_window_buffer(data, valid_count)
    %#codegen

    window_size = 1000;
    channels = 3;

    persistent buffer idx

    if isempty(buffer)
        buffer = zeros(window_size, channels);
        idx = 0;
    end

    for i = 1:valid_count
        if idx < window_size
            idx = idx + 1;
            buffer(idx, :) = data(i, :);
        else
            buffer(1:end-1, :) = buffer(2:end, :);
            buffer(end, :) = data(i, :);
        end
    end

    window_out = buffer;
    is_ready = (idx >= window_size);
end

== matlab function EMG_DR_E2E_pipeline_simulink/Classfication and Execution/Drone Execution/Angle converter ==
  data: T input; w12 output; t1 input; t2 input; t3 input; w22 output; w32 output; w42 output
function [w12,w22,w32,w42]  = fcn(T,t1,t2,t3)

d=0.176777;ct=8.586e-08;cq=4.81e-09;
A=[ct ct ct ct; -(d*ct) (d*ct) (d*ct) -(d*ct); -d*ct -d*ct d*ct d*ct;-cq cq -cq cq];
B=[T t1*1.414 t2*1.414 t3]';
C=inv(A)*B;

w12=C(1,1);
w22=C(2,1);w32=C(3,1);w42=C(4,1);

if(w12<0)
    w12=0;
end
if(w22<0)
    w22=0;
end
if(w32<0)
    w32=0;
end
if(w42<0)
    w42=0;
end

== matlab function EMG_DR_E2E_pipeline_simulink/Classfication and Execution/Drone Execution/MATLAB Function ==
  data: gesture_idx input; drone_idx output
function drone_idx = ges2drone(gesture_idx)
    persistent past_gest
    persistent change_gest
    if isempty(past_gest)
        past_gest = 0;
        change_gest = true;
    end
    
    if change_gest
        if gesture_idx == 8    % NaN
            if past_gest > 0
                drone_idx = past_gest;
            else
                drone_idx = 0;
            end
        else
            if gesture_idx == 7  
                drone_idx = gesture_idx;
                past_gest = drone_idx;
            else
                drone_idx = gesture_idx;
                past_gest = drone_idx;
                change_gest = false;
            end
            
        end
 
    else
        if gesture_idx == 7
            drone_idx = gesture_idx;
            past_gest = drone_idx;
            change_gest = true;
        else
            drone_idx = past_gest;
        end
    end
end
